simulink model "lab_3_scheme"  (R2021b)
settings: Solver=VariableStepAuto  StartTime=0.0  StopTime=0.2  RelTol=1e-3
values from neighbouring files (symbols this model uses):
  Jn = 2*Jd    (= 0.000334)    [lab_3_script.m]
  Kd = place(SYS.A,SYS.B,pd)    [lab_3_script.m]
  ke = (Un-R*In)/wn    (= 0.320333333333)    [lab_3_script.m]
  km = Mn/In    (= 0.228971962617)    [lab_3_script.m]
  ku = 20    [lab_3_script.m]
  L = l'    [lab_3_script.m]
  R = 8.5    [lab_3_script.m]
  SYS = ss(Ad,Bd,Cd,Dd,Ts)    [lab_3_script.m]
  Ts = 0.001    [lab_3_script.m]
settings Model: Creator=vkad  LastModifiedBy=vkad

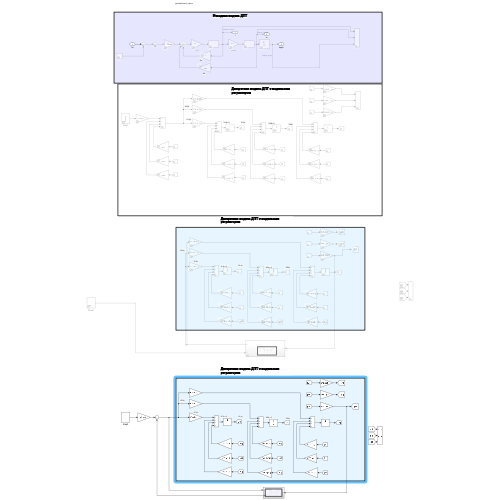
[thumbnail: Simulink's stored preview of the top-level diagram]
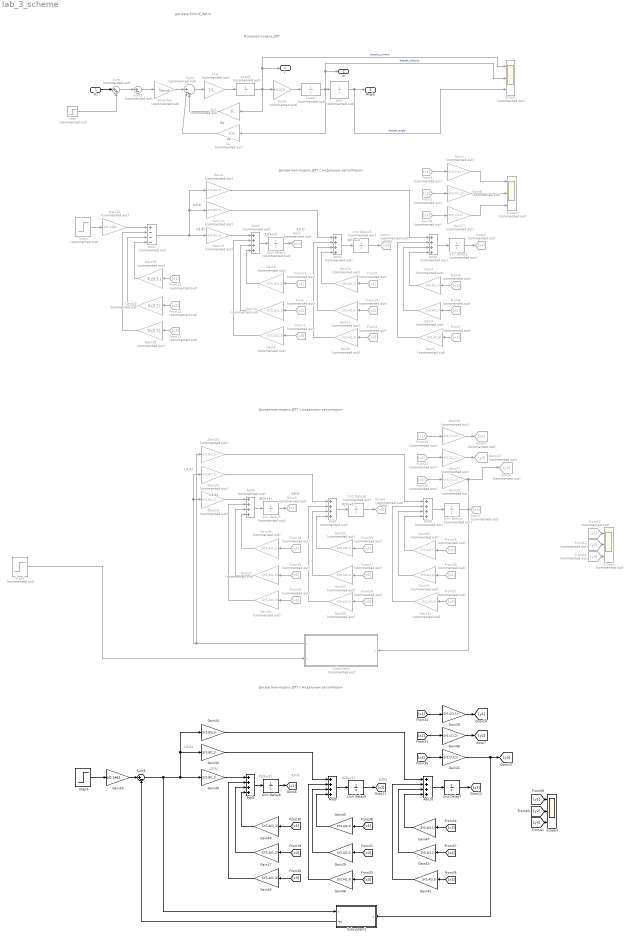
== system lab_3_scheme ==
  note: Исходная модель ДПТ
  note: Gain4
  note: get data from tf_dpt.m
  note: kе
  note: Rя
  note: Дискретная модель ДПТ с модальным регулятором
  note: U2(k)
  note: U1(k)
  note: X2(k+1)
  note: X1(k+1)
  note: X2(k)
  note: X1(k)
  note: Дискретная модель ДПТ с модальным регулятором
  note: U2(k)
  note: U1(k)
  note: X2(k+1)
  note: X1(k+1)
  note: X2(k)
  note: X1(k)
  note: Дискретная модель ДПТ с модальным регулятором
  note: U2(k)
  note: U1(k)
  note: X2(k+1)
  note: X1(k+1)
  note: X2(k)
  note: X1(k)
  Uz : Inport
  1/Lя : Gain  Commented=on  Gain=1/L
  Add1 : Sum  Commented=on  Inputs=+---
  Add10 : Sum  Inputs=++++
  Add{2..4,6..8} (6 alike) : Sum  Commented=on  Inputs=++++
  Add5 : Sum  Inputs=++++
  Add9 : Sum  Inputs=++++
  Amplifier : Gain  Commented=on  Gain=ku
  Ce : Gain  Commented=on  Gain=ke
  Ce1 : Gain  Commented=on  Gain=R
  From{,2,8,10,12,15,17,22,28} (9 alike) : From  Commented=on  GotoTag=x2
  From{1,4,6..7,13,16,24,26..27} (9 alike) : From  Commented=on  GotoTag=x3
  From{3,5,9,11,14,18,23,25,29} (9 alike) : From  Commented=on  GotoTag=x1
  From42 : From  Commented=on  GotoTag=y1
  From43 : From  Commented=on  GotoTag=y2
  From44 : From  Commented=on  GotoTag=y3
  Gain1 : Gain  Commented=on  Gain=SYS.C(1,1)
  Gain10 : Gain  Commented=on  Gain=SYS.A(1,2)
  Gain11 : Gain  Commented=on  Gain=SYS.A(2,2)
  Gain12 : Gain  Commented=on  Gain=SYS.B(2,1)
  Gain13 : Gain  Commented=on  Gain=SYS.B(1,1)
  Gain14 : Gain  Commented=on  Gain=SYS.A(2,1)
  Gain15 : Gain  Commented=on  Gain=1/0.1462
  Gain16 : Gain  Commented=on  Gain=Kd(2)
  Gain17 : Gain  Commented=on  Gain=SYS.C(3,3)
  Gain18 : Gain  Commented=on  Gain=Kd(3)
  Gain19 : Gain  Commented=on  Gain=Kd(1)
  Gain2 : Gain  Commented=on  Gain=SYS.A(3,3)
  Gain20 : Gain  Commented=on  Gain=SYS.C(1,1)
  Gain21 : Gain  Commented=on  Gain=SYS.A(1,2)
  Gain22 : Gain  Commented=on  Gain=SYS.A(2,2)
  Gain23 : Gain  Commented=on  Gain=SYS.B(2,1)
  Gain24 : Gain  Commented=on  Gain=SYS.B(1,1)
  Gain25 : Gain  Commented=on  Gain=SYS.A(2,1)
  Gain26 : Gain  Gain=SYS.C(1,1)
  Gain27 : Gain  Gain=SYS.A(1,2)
  Gain28 : Gain  Commented=on  Gain=SYS.C(3,3)
  Gain29 : Gain  Gain=SYS.A(2,2)
  Gain3 : Gain  Commented=on  Gain=SYS.A(3,2)
  Gain30 : Gain  Gain=SYS.B(2,1)
  Gain31 : Gain  Commented=on  Gain=SYS.A(3,3)
  Gain32 : Gain  Commented=on  Gain=SYS.A(3,2)
  Gain33 : Gain  Commented=on  Gain=SYS.B(3,1)
  Gain34 : Gain  Commented=on  Gain=SYS.A(1,3)
  Gain35 : Gain  Commented=on  Gain=SYS.A(2,3)
  Gain36 : Gain  Commented=on  Gain=SYS.A(3,1)
  Gain37 : Gain  Commented=on  Gain=SYS.C(2,2)
  Gain38 : Gain  Commented=on  Gain=SYS.A(1,1)
  Gain39 : Gain  Gain=SYS.B(1,1)
  Gain4 : Gain  Commented=on  Gain=SYS.B(3,1)
  Gain40 : Gain  Gain=SYS.A(2,1)
  Gain41 : Gain  Gain=SYS.C(3,3)
  Gain42 : Gain  Gain=SYS.A(3,3)
  Gain43 : Gain  Gain=SYS.A(3,2)
  Gain44 : Gain  Gain=SYS.B(3,1)
  Gain45 : Gain  Gain=SYS.A(1,3)
  Gain46 : Gain  Gain=SYS.A(2,3)
  Gain47 : Gain  Gain=SYS.A(3,1)
  Gain48 : Gain  Gain=SYS.C(2,2)
  Gain49 : Gain  Gain=SYS.A(1,1)
  Gain5 : Gain  Commented=on  Gain=SYS.A(1,3)
  Gain50 : Gain  Gain=1/0.1462
  Gain6 : Gain  Commented=on  Gain=SYS.A(2,3)
  Gain7 : Gain  Commented=on  Gain=SYS.A(3,1)
  Gain8 : Gain  Commented=on  Gain=SYS.C(2,2)
  Gain9 : Gain  Commented=on  Gain=SYS.A(1,1)
  Goto : Goto  Commented=on  GotoTag=x1
  Goto1 : Goto  Commented=on  GotoTag=x2
  Goto10 : Goto  Commented=on  GotoTag=y2
  Goto2 : Goto  Commented=on  GotoTag=x3
  Goto3 : Goto  Commented=on  GotoTag=x1
  Goto4 : Goto  Commented=on  GotoTag=x2
  Goto5 : Goto  Commented=on  GotoTag=x3
  Goto6 : Goto  Commented=on  GotoTag=y3
  Goto9 : Goto  Commented=on  GotoTag=y1
  Load1 : TransferFcn  Commented=on  Denominator=[1 0]
  Load2 : TransferFcn  Commented=on  Denominator=[1 0]
  Scope : Scope  Commented=on  NumInputPorts=3
  Scope1 : Scope  Commented=on  NumInputPorts=3
  Scope2 : Scope  Commented=on  NumInputPorts=3
  Scope3 : Scope  NumInputPorts=3
  Step : Step  Commented=on  Time=0  SampleTime=0
  Step1 : Step  Commented=on  Time=0  SampleTime=0
  Step2 : Step  Commented=on  Time=0  SampleTime=0
  Step3 : Step  Time=0  SampleTime=0
  Subsystem : Subsystem  Commented=on
      settings: PortSchema="{\"entries\":[{\"content\":{\"sides\":[{\"content\":{\"connectorIds\":[\"Out1\",\"In1\"]},\"type\":\"ConnectorPlacement.EquallySpacedRectSide\",\"uuid\":\"1ae5a343-437d-4cb9-9822-e2db9fa7010c\"},{\"content\":{\"connectorIds\":[\"In2\"],\"side\":\"RIGHT\"},\"type\":\"ConnectorPlacement.EquallySpacedRectSide\",\"uuid\":\"a13fd255-885b-49a4-bdfe-42517e7d2bb6\"},{\"content\":{\"connectorIds\":[],\"side\":\"TOP\"},\"type\":\"ConnectorPlacement.EquallySpacedRectSide\",\"uuid\":\"ec77d7e4-a70f-42b2-8285-e16af54c9a8e\"}]},\"type\":\"ConnectorPlacement.EquallySpacedConnector\",\"uuid\":\"a53451af-0313-4fad-91e1-dbe8374f8c5a\"}],\"packageUris\":[\"http://schema.mathworks.com/mf0/Connector/R2020b\"],\"version\":\"1.0\"}"
  Subsystem1 : Subsystem
      settings: PortSchema="{\"entries\":[{\"content\":{\"sides\":[{\"content\":{\"connectorIds\":[\"In1\",\"Out1\"]},\"type\":\"ConnectorPlacement.EquallySpacedRectSide\",\"uuid\":\"1ae5a343-437d-4cb9-9822-e2db9fa7010c\"},{\"content\":{\"connectorIds\":[\"In2\"],\"side\":\"RIGHT\"},\"type\":\"ConnectorPlacement.EquallySpacedRectSide\",\"uuid\":\"a13fd255-885b-49a4-bdfe-42517e7d2bb6\"},{\"content\":{\"connectorIds\":[],\"side\":\"TOP\"},\"type\":\"ConnectorPlacement.EquallySpacedRectSide\",\"uuid\":\"ec77d7e4-a70f-42b2-8285-e16af54c9a8e\"}]},\"type\":\"ConnectorPlacement.EquallySpacedConnector\",\"uuid\":\"a53451af-0313-4fad-91e1-dbe8374f8c5a\"}],\"packageUris\":[\"http://schema.mathworks.com/mf0/Connector/R2020b\"],\"version\":\"1.0\"}"
  Sum : Sum  Commented=on  Inputs=|++
  Sum1 : Sum  Commented=on  Inputs=||+--
  Sum2 : Sum  Commented=on  Inputs=|+-
  Sum5 : Sum  Inputs=|+-
  Unit Delay{1..6} (6 alike) : UnitDelay  Commented=on  SampleTime=Ts  HasFrameUpgradeWarning=on
  Unit Delay7 : UnitDelay  SampleTime=Ts  HasFrameUpgradeWarning=on
  Unit Delay8 : UnitDelay  SampleTime=Ts  HasFrameUpgradeWarning=on
  Unit Delay9 : UnitDelay  SampleTime=Ts  HasFrameUpgradeWarning=on
  gear : TransferFcn  Commented=on  Numerator=1  Denominator=[1 0]
  Км/Jн : Gain  Commented=on  Gain=km/Jn
  I : Outport
  w : Outport  Port=2
  Angle : Outport  Port=3
  wires:
  Amplifier/1 -> Sum1/1
  1/Lя/1 -> Load1/1
  Sum/1 -> Sum2/1
  Sum2/1 -> Amplifier/1
  gear/1 -> Scope/3, Angle/1  "bessel_angle"
  Км/Jн/1 -> Load2/1
  Load2/1 -> Scope/2, w/1, Ce/1, gear/1  "bessel_velosity"
  Step/1 -> Sum/2
  Load1/1 -> Ce1/1, Км/Jн/1, Scope/1, I/1  "bessel_current"
  Sum1/1 -> 1/Lя/1
  Ce/1 -> Sum1/2
  Uz/1 -> Sum/1
  Ce1/1 -> Sum1/3
  Gain13/1 -> Add2/1
  Add3/1 -> Unit Delay3/1
  Gain9/1 -> Add2/4
  Gain10/1 -> Add2/3
  Unit Delay3/1 -> Goto1/1
  Gain12/1 -> Add3/1
  Add2/1 -> Unit Delay2/1
  Unit Delay2/1 -> Goto/1
  Unit Delay1/1 -> Goto2/1
  Add4/1 -> Unit Delay1/1
  Gain2/1 -> Add4/2
  Gain4/1 -> Add4/1
  Gain7/1 -> Add4/4
  Gain1/1 -> Scope2/1
  Gain8/1 -> Scope2/2
  From/1 -> Gain10/1
  From1/1 -> Gain5/1
  From2/1 -> Gain8/1
  From3/1 -> Gain1/1
  From4/1 -> Gain6/1
  From5/1 -> Gain7/1
  From6/1 -> Gain17/1
  From7/1 -> Gain2/1
  From8/1 -> Gain3/1
  Gain3/1 -> Add4/3
  From9/1 -> Gain14/1
  Gain6/1 -> Add3/2
  Gain11/1 -> Add3/3
  Gain14/1 -> Add3/4
  From10/1 -> Gain11/1
  From11/1 -> Gain9/1
  Gain5/1 -> Add2/2
  Add1/1 -> Gain4/1, Gain12/1, Gain13/1
  Step1/1 -> Gain15/1
  From14/1 -> Gain19/1
  From13/1 -> Gain18/1
  From12/1 -> Gain16/1
  Gain17/1 -> Scope2/3
  Gain15/1 -> Add1/1
  Gain18/1 -> Add1/2
  Gain16/1 -> Add1/3
  Gain19/1 -> Add1/4
  Gain34/1 -> Add6/2
  From18/1 -> Gain38/1
  From17/1 -> Gain22/1
  Gain25/1 -> Add7/4
  Gain22/1 -> Add7/3
  Gain35/1 -> Add7/2
  From29/1 -> Gain25/1
  Gain32/1 -> Add8/3
  From28/1 -> Gain32/1
  From27/1 -> Gain31/1
  From26/1 -> Gain28/1
  From25/1 -> Gain36/1
  From24/1 -> Gain35/1
  From23/1 -> Gain20/1
  From22/1 -> Gain37/1
  From16/1 -> Gain34/1
  From15/1 -> Gain21/1
  Gain37/1 -> Goto10/1
  Gain20/1 -> Goto9/1
  Gain36/1 -> Add8/4
  Gain33/1 -> Add8/1
  Gain31/1 -> Add8/2
  Add8/1 -> Unit Delay4/1
  Unit Delay4/1 -> Goto5/1
  Unit Delay5/1 -> Goto3/1
  Add6/1 -> Unit Delay5/1
  Gain23/1 -> Add7/1
  Unit Delay6/1 -> Goto4/1
  Gain21/1 -> Add6/3
  Gain38/1 -> Add6/4
  Add7/1 -> Unit Delay6/1
  Gain24/1 -> Add6/1
  From42/1 -> Scope1/1
  From43/1 -> Scope1/2
  From44/1 -> Scope1/3
  Subsystem/1(u) -> Gain23/1, Gain24/1, Gain33/1
  Gain28/1 -> Goto6/1, Subsystem/2(y)
  Step2/1 -> Subsystem/1(in)
  [y3] -> Scope3/3
  [y2] -> Scope3/2
  [y1] -> Scope3/1
  Gain39/1 -> Add5/1
  Add9/1 -> Unit Delay9/1
  Gain49/1 -> Add5/4
  Gain27/1 -> Add5/3
  Unit Delay9/1 -> [x2]
  Gain30/1 -> Add9/1
  Add5/1 -> Unit Delay8/1
  Unit Delay8/1 -> [x1]
  Unit Delay7/1 -> [x3]
  Add10/1 -> Unit Delay7/1
  Gain42/1 -> Add10/2
  Gain44/1 -> Add10/1
  Gain47/1 -> Add10/4
  Gain26/1 -> [y1]
  Gain48/1 -> [y2]
  [x2] -> Gain27/1
  [x3] -> Gain45/1
  [x2] -> Gain48/1
  [x1] -> Gain26/1
  [x3] -> Gain46/1
  [x1] -> Gain47/1
  [x3] -> Gain41/1
  [x3] -> Gain42/1
  [x2] -> Gain43/1
  Gain43/1 -> Add10/3
  [x1] -> Gain40/1
  Gain46/1 -> Add9/2
  Gain29/1 -> Add9/3
  Gain40/1 -> Add9/4
  [x2] -> Gain29/1
  [x1] -> Gain49/1
  Gain45/1 -> Add5/2
  Step3/1 -> Gain50/1
  Gain50/1 -> Sum5/1
  Gain41/1 -> Subsystem1/2(y), [y3]
  Sum5/1 -> Subsystem1/1(u), Gain44/1, Gain30/1, Gain39/1
  Subsystem1/1(reg) -> Sum5/2

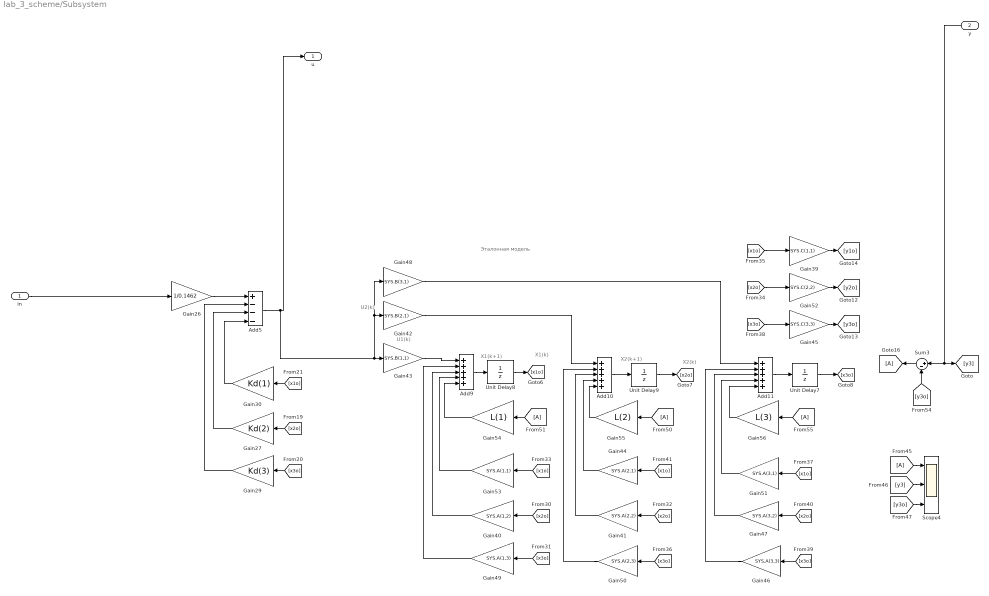
== system lab_3_scheme/Subsystem ==
  note: U2(k)
  note: U1(k)
  note: X2(k+1)
  note: X1(k+1)
  note: X2(k)
  note: X1(k)
  note: Эталонная модель
  in : Inport
  y : Inport  Port=2
  Add10 : Sum  Inputs=+++++
  Add11 : Sum  Inputs=+++++
  Add5 : Sum  Inputs=+---
  Add9 : Sum  Inputs=+++++
  Gain26 : Gain  Gain=1/0.1462
  Gain27 : Gain  Gain=Kd(2)
  Gain29 : Gain  Gain=Kd(3)
  Gain30 : Gain  Gain=Kd(1)
  Gain39 : Gain  Gain=SYS.C(1,1)
  Gain40 : Gain  Gain=SYS.A(1,2)
  Gain41 : Gain  Gain=SYS.A(2,2)
  Gain42 : Gain  Gain=SYS.B(2,1)
  Gain43 : Gain  Gain=SYS.B(1,1)
  Gain44 : Gain  Gain=SYS.A(2,1)
  Gain45 : Gain  Gain=SYS.C(3,3)
  Gain46 : Gain  Gain=SYS.A(3,3)
  Gain47 : Gain  Gain=SYS.A(3,2)
  Gain48 : Gain  Gain=SYS.B(3,1)
  Gain49 : Gain  Gain=SYS.A(1,3)
  Gain50 : Gain  Gain=SYS.A(2,3)
  Gain51 : Gain  Gain=SYS.A(3,1)
  Gain52 : Gain  Gain=SYS.C(2,2)
  Gain53 : Gain  Gain=SYS.A(1,1)
  Gain54 : Gain  Gain=L(1)
  Gain55 : Gain  Gain=L(2)
  Gain56 : Gain  Gain=L(3)
  Scope4 : Scope  NumInputPorts=3
  Sum3 : Sum  Inputs=|+-
  Unit Delay7 : UnitDelay  SampleTime=Ts  HasFrameUpgradeWarning=on
  Unit Delay8 : UnitDelay  SampleTime=Ts  HasFrameUpgradeWarning=on
  Unit Delay9 : UnitDelay  SampleTime=Ts  HasFrameUpgradeWarning=on
  u : Outport
  wires:
  [x3o] -> Gain50/1
  [x3o] -> Gain29/1
  Gain40/1 -> Add9/3
  Sum3/1 -> [A]
  Unit Delay9/1 -> [x2o]
  Gain45/1 -> [y3o]
  Gain43/1 -> Add9/1
  Gain29/1 -> Add5/2
  Add9/1 -> Unit Delay8/1
  Gain54/1 -> Add9/5
  Add10/1 -> Unit Delay9/1
  Gain39/1 -> [y1o]
  Gain42/1 -> Add10/1
  Add11/1 -> Unit Delay7/1
  [x1o] -> Gain30/1
  Gain44/1 -> Add10/4
  [x2o] -> Gain52/1
  Add5/1 -> Gain48/1, Gain42/1, Gain43/1, u/1
  Gain46/1 -> Add11/2
  Gain27/1 -> Add5/3
  [A] -> Gain55/1
  [x2o] -> Gain47/1
  y/1 -> [y3], Sum3/1
  Gain48/1 -> Add11/1
  [x1o] -> Gain51/1
  Gain49/1 -> Add9/2
  [x2o] -> Gain27/1
  [x2o] -> Gain41/1
  [x3o] -> Gain49/1
  Gain55/1 -> Add10/5
  Unit Delay8/1 -> [x1o]
  [x1o] -> Gain44/1
  [x1o] -> Gain53/1
  [A] -> Gain56/1
  Gain30/1 -> Add5/4
  Gain52/1 -> [y2o]
  Gain51/1 -> Add11/4
  [x3o] -> Gain46/1
  [x1o] -> Gain39/1
  in/1 -> Gain26/1
  [A] -> Gain54/1
  [x2o] -> Gain40/1
  Gain50/1 -> Add10/2
  Gain56/1 -> Add11/5
  Gain47/1 -> Add11/3
  Gain41/1 -> Add10/3
  Unit Delay7/1 -> [x3o]
  [x3o] -> Gain45/1
  Gain53/1 -> Add9/4
  [y3o] -> Sum3/2
  Gain26/1 -> Add5/1
  [A] -> Scope4/1
  [y3o] -> Scope4/3
  [y3] -> Scope4/2

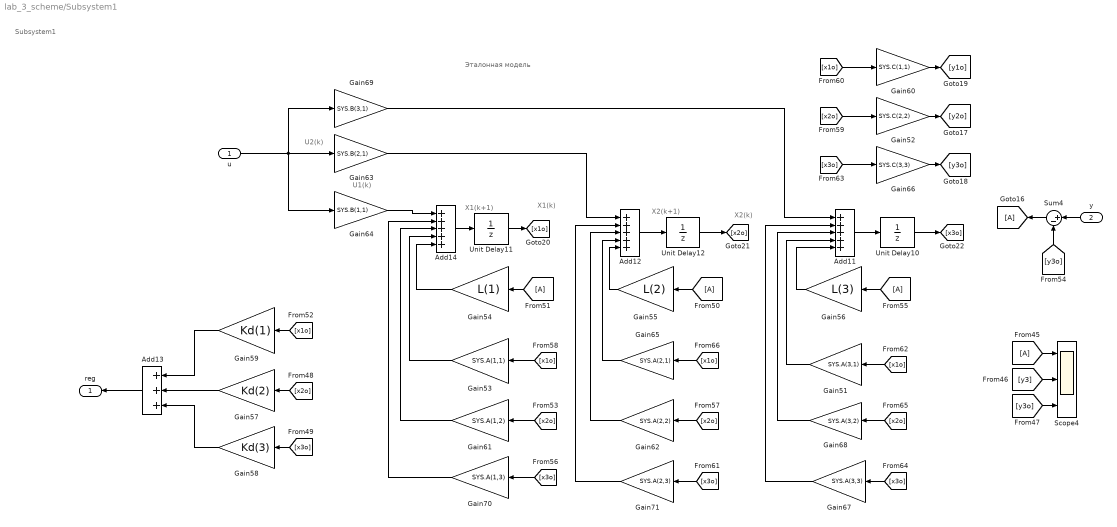
== system lab_3_scheme/Subsystem1 ==
  note: Subsystem1
  note: U2(k)
  note: U1(k)
  note: X2(k+1)
  note: X1(k+1)
  note: X2(k)
  note: X1(k)
  note: Эталонная модель
  u : Inport
  y : Inport  Port=2
  Add11 : Sum  Inputs=+++++
  Add12 : Sum  Inputs=+++++
  Add13 : Sum  Inputs=+++
  Add14 : Sum  Inputs=+++++
  Gain51 : Gain  Gain=SYS.A(3,1)
  Gain52 : Gain  Gain=SYS.C(2,2)
  Gain53 : Gain  Gain=SYS.A(1,1)
  Gain54 : Gain  Gain=L(1)
  Gain55 : Gain  Gain=L(2)
  Gain56 : Gain  Gain=L(3)
  Gain57 : Gain  Gain=Kd(2)
  Gain58 : Gain  Gain=Kd(3)
  Gain59 : Gain  Gain=Kd(1)
  Gain60 : Gain  Gain=SYS.C(1,1)
  Gain61 : Gain  Gain=SYS.A(1,2)
  Gain62 : Gain  Gain=SYS.A(2,2)
  Gain63 : Gain  Gain=SYS.B(2,1)
  Gain64 : Gain  Gain=SYS.B(1,1)
  Gain65 : Gain  Gain=SYS.A(2,1)
  Gain66 : Gain  Gain=SYS.C(3,3)
  Gain67 : Gain  Gain=SYS.A(3,3)
  Gain68 : Gain  Gain=SYS.A(3,2)
  Gain69 : Gain  Gain=SYS.B(3,1)
  Gain70 : Gain  Gain=SYS.A(1,3)
  Gain71 : Gain  Gain=SYS.A(2,3)
  Scope4 : Scope  NumInputPorts=3
  Sum4 : Sum  Inputs=|+-
  Unit Delay10 : UnitDelay  SampleTime=Ts  HasFrameUpgradeWarning=on
  Unit Delay11 : UnitDelay  SampleTime=Ts  HasFrameUpgradeWarning=on
  Unit Delay12 : UnitDelay  SampleTime=Ts  HasFrameUpgradeWarning=on
  reg : Outport
  wires:
  u/1 -> Gain69/1, Gain64/1, Gain63/1
  [x1o] -> Gain65/1
  Gain53/1 -> Add14/4
  [y3] -> Scope4/2
  [y3o] -> Sum4/2
  Gain69/1 -> Add11/1
  [A] -> Scope4/1
  [x2o] -> Gain68/1
  Gain61/1 -> Add14/3
  Gain63/1 -> Add12/1
  Gain60/1 -> [y1o]
  [y3o] -> Scope4/3
  [x3o] -> Gain70/1
  [x2o] -> Gain61/1
  Gain67/1 -> Add11/2
  Add11/1 -> Unit Delay10/1
  [A] -> Gain55/1
  Gain54/1 -> Add14/5
  Sum4/1 -> [A]
  Unit Delay10/1 -> [x3o]
  y/1 -> Sum4/1
  [x1o] -> Gain51/1
  [x3o] -> Gain67/1
  [x1o] -> Gain59/1
  Gain70/1 -> Add14/2
  Gain55/1 -> Add12/5
  [x2o] -> Gain62/1
  [x2o] -> Gain57/1
  Unit Delay11/1 -> [x1o]
  [x1o] -> Gain53/1
  Unit Delay12/1 -> [x2o]
  [A] -> Gain56/1
  [x1o] -> Gain60/1
  Gain51/1 -> Add11/4
  Gain52/1 -> [y2o]
  Gain71/1 -> Add12/2
  [A] -> Gain54/1
  [x2o] -> Gain52/1
  Gain56/1 -> Add11/5
  Gain62/1 -> Add12/3
  Gain68/1 -> Add11/3
  [x3o] -> Gain71/1
  [x3o] -> Gain58/1
  Gain66/1 -> [y3o]
  Gain64/1 -> Add14/1
  Add14/1 -> Unit Delay11/1
  Add12/1 -> Unit Delay12/1
  Gain65/1 -> Add12/4
  [x3o] -> Gain66/1
  Add13/1 -> reg/1
  Gain59/1 -> Add13/1
  Gain57/1 -> Add13/2
  Gain58/1 -> Add13/3
